simulink model "lab3p2"  (R2023b)
settings: Solver=ode3  StartTime=0.0  StopTime=Tmdl  FixedStep=To/100  RelTol=1e-3
undefined symbols (not defined in the file or in its folder): an, dsc, To
settings Model: Creator=deniskirbaba  LastModifiedBy=Максим

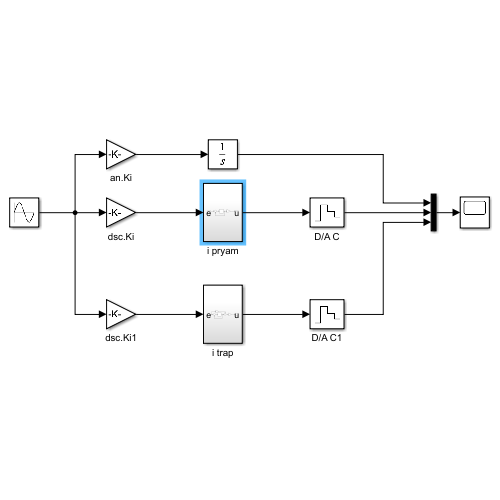
[thumbnail: Simulink's stored preview of the top-level diagram]
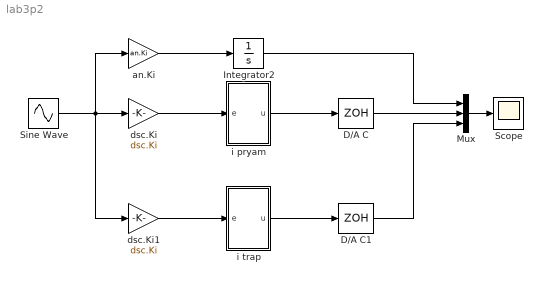
== system lab3p2 ==
  D/A C : ZeroOrderHold  SampleTime=To
  D/A C1 : ZeroOrderHold  SampleTime=To
  Integrator2 : Integrator
  Mux : Mux  Inputs=3
  Scope : Scope
  Sine Wave : Sin  Frequency=2*pi  SampleTime=0
  an.Ki : Gain  Gain=an.Ki
  dsc.Ki : Gain  Gain=dsc.Ki
  dsc.Ki1 : Gain  Gain=dsc.Ki
  i pryam : Subsystem
  i trap : Subsystem
  wires:
  an.Ki/1 -> Integrator2/1
  D/A C/1 -> Mux/2
  Mux/1 -> Scope/1
  Integrator2/1 -> Mux/1
  Sine Wave/1 -> an.Ki/1, dsc.Ki1/1, dsc.Ki/1
  D/A C1/1 -> Mux/3
  dsc.Ki/1 -> i pryam/1(e)
  i pryam/1(u) -> D/A C/1
  dsc.Ki1/1 -> i trap/1(e)
  i trap/1(u) -> D/A C1/1

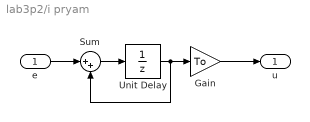
== system lab3p2/i pryam ==
  e : Inport
  Gain : Gain  Gain=To
  Sum : Sum  Inputs=|++
  Unit Delay : UnitDelay  SampleTime=To  HasFrameUpgradeWarning=on
  u : Outport
  wires:
  Sum/1 -> Unit Delay/1
  Unit Delay/1 -> Sum/2, Gain/1
  e/1 -> Sum/1
  Gain/1 -> u/1

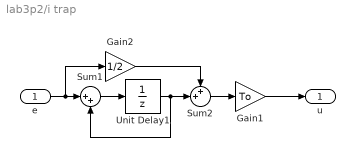
== system lab3p2/i trap ==
  e : Inport
  Gain1 : Gain  Gain=To
  Gain2 : Gain  Gain=1/2
  Sum1 : Sum  Inputs=|++
  Sum2 : Sum  Inputs=++|
  Unit Delay1 : UnitDelay  SampleTime=To  HasFrameUpgradeWarning=on
  u : Outport
  wires:
  Unit Delay1/1 -> Sum2/2, Sum1/2
  Sum2/1 -> Gain1/1
  Gain2/1 -> Sum2/1
  Sum1/1 -> Unit Delay1/1
  e/1 -> Gain2/1, Sum1/1
  Gain1/1 -> u/1
